simulink model "e02"  (R2023b)
settings: Solver=VariableStepAuto  StartTime=0.0  StopTime=10.0  RelTol=1e-3
values from neighbouring files (symbols this model uses):
  A = [0, 1, 0, 0 ... (first row only)    [e01.m]
  B = [0, 0 ... (first row only)    [e01.m]
  C = [1, 0, 0, 0 ... (first row only)    [e01.m]
  D = [0, 0 ... (first row only)    [e01.m]
settings Model: Creator=jitbi  LastModifiedBy=jitbi

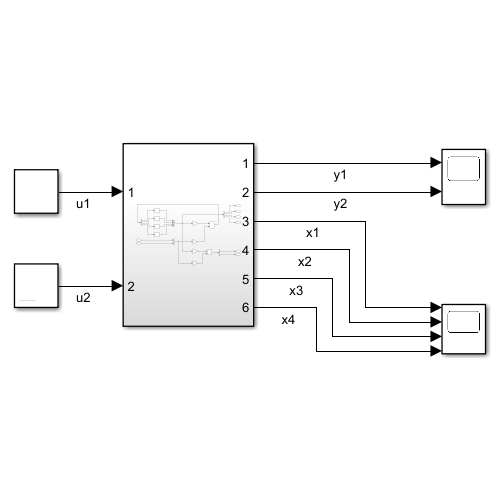
[thumbnail: Simulink's stored preview of the top-level diagram]
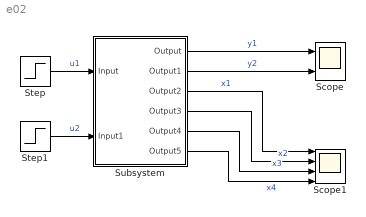
== system e02 ==
  Scope : Scope  NumInputPorts=2
  Scope1 : Scope  NumInputPorts=4
  Step : Step  Time=0  SampleTime=1e-6
  Step1 : Step  Time=0  SampleTime=1e-6
  Subsystem : Subsystem
  wires:
  Step/1 -> Subsystem/1(Input)  "u1"
  Step1/1 -> Subsystem/2(Input1)  "u2"
  Subsystem/1(Output) -> Scope/1  "y1"
  Subsystem/2(Output1) -> Scope/2  "y2"
  Subsystem/3(Output2) -> Scope1/1  "x1"
  Subsystem/4(Output3) -> Scope1/2  "x2"
  Subsystem/5(Output4) -> Scope1/3  "x3"
  Subsystem/6(Output5) -> Scope1/4  "x4"

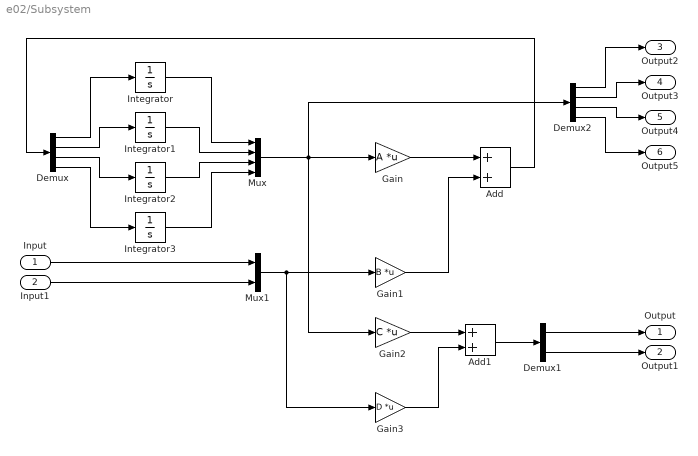
== system e02/Subsystem ==
  Input : Inport
  Input1 : Inport  Port=2
  Add : Sum
  Add1 : Sum
  Demux : Demux
  Demux1 : Demux  Outputs=2
  Demux2 : Demux
  Gain : Gain  Gain=A  Multiplication=Matrix(K*u)
  Gain1 : Gain  Gain=B  Multiplication=Matrix(K*u)
  Gain2 : Gain  Gain=C  Multiplication=Matrix(K*u)
  Gain3 : Gain  Gain=D  Multiplication=Matrix(K*u)
  Integrator{,1..3} (4 alike) : Integrator
  Mux : Mux
  Mux1 : Mux  Inputs=2
  Output : Outport
  Output1 : Outport  Port=2
  Output2 : Outport  Port=3
  Output3 : Outport  Port=4
  Output4 : Outport  Port=5
  Output5 : Outport  Port=6
  wires:
  Demux2/1 -> Output2/1
  Mux1/1 -> Gain3/1, Gain1/1
  Gain1/1 -> Add/2
  Demux1/1 -> Output/1
  Demux2/2 -> Output3/1
  Integrator/1 -> Mux/1
  Add/1 -> Demux/1
  Gain/1 -> Add/1
  Mux/1 -> Demux2/1, Gain2/1, Gain/1
  Input/1 -> Mux1/1
  Input1/1 -> Mux1/2
  Demux2/3 -> Output4/1
  Demux/2 -> Integrator1/1
  Integrator1/1 -> Mux/2
  Demux/3 -> Integrator2/1
  Integrator2/1 -> Mux/3
  Demux/4 -> Integrator3/1
  Integrator3/1 -> Mux/4
  Demux/1 -> Integrator/1
  Demux2/4 -> Output5/1
  Gain3/1 -> Add1/2
  Add1/1 -> Demux1/1
  Gain2/1 -> Add1/1
  Demux1/2 -> Output1/1
